simulink model "acc_PV"  (R2021b)
settings: Solver=FixedStepAuto  StartTime=0.0  StopTime=40  FixedStep=0.0005  RelTol=1e-3
undefined symbols (not defined in the file or in its folder): sigbuilder_block
libraries: Solver_SF x1
settings Model: Creator=power  LastModifiedBy=power
settings DataIOCC: ReturnWorkspaceOutputs=off

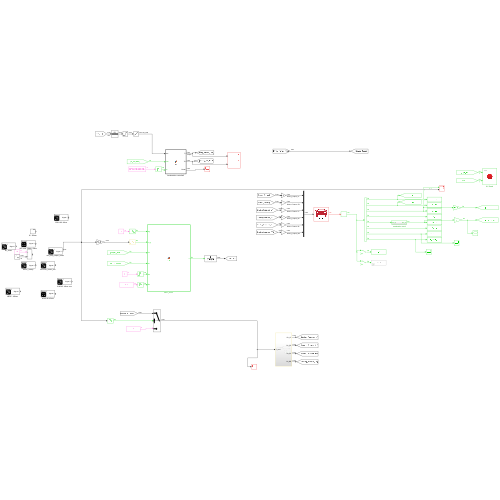
[thumbnail: Simulink's stored preview of the top-level diagram]
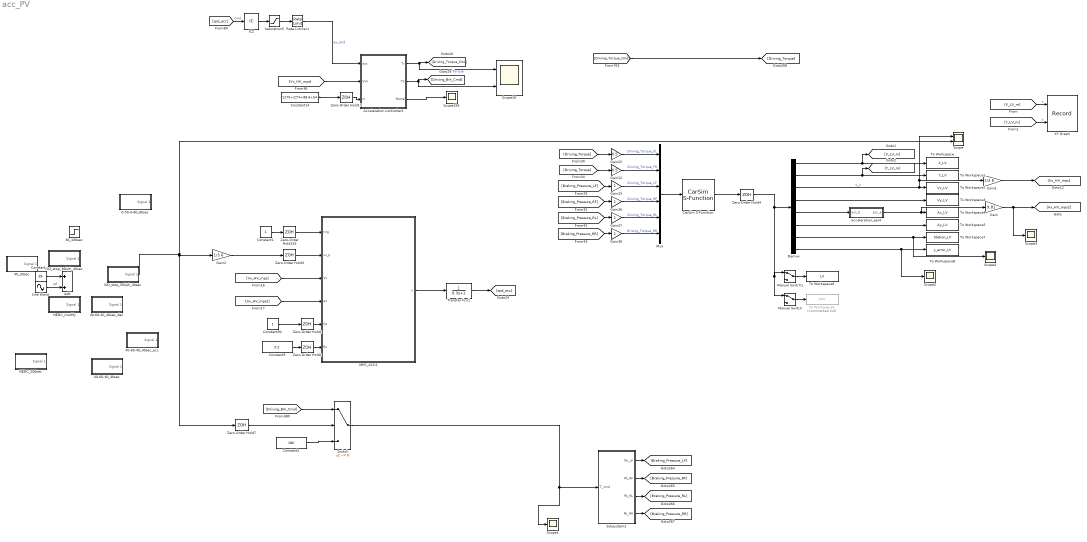
== system acc_PV ==
  0-50-0-80_80sec : Subsystem  Tag=STV Subsys  LoadFcn=sigbuilder_block('load');  StartFcn=sigbuilder_block('start');  StopFcn=sigbuilder_block('stop');  ClipboardFcn=sigbuilder_block('clipboard');  mask(Sigbuilder block){tuvar=[0:10]}
      mask help: Simulink:masks:SigbuilderBlock_MD
      mask init:
      | if ~strcmp(get_param(bdroot(gcbh),'SimulationStatus'),'stopped') tuvar = sigbuilder_block('maskInit'); end
      settings: CopyFcn=sigbuilder_block('copy');  DeleteFcn=sigbuilder_block('delete');  ModelCloseFcn=sigbuilder_block('modelClose');  PreSaveFcn=sigbuilder_block('preSave');  PauseFcn=sigbuilder_block('pause');  ContinueFcn=sigbuilder_block('continue');  NameChangeFcn=sigbuilder_block('namechange');  OpenFcn=sigbuilder_block('open',[523.8 -84 622.8 385.8 ]);  CloseFcn=sigbuilder_block('close');
      mask Display: plot(0, 0, 100, 100,[2, 2, 32, 32, 2], [68, 8, 8, 68, 68],[32, 2], [38, 38], [32, 19, 2],[53, 60, 44], [32, 17, 17, 2],[16, 16, 31, 31]);txt = getActiveGroup(gcbh);text(2, 100, txt,'verticalAlignment', 'top');
  36_100sec : Step  Time=0  Before=28  After=28  SampleTime=0
  40-60-40_40sec : Subsystem  Tag=STV Subsys  LoadFcn=sigbuilder_block('load');  StartFcn=sigbuilder_block('start');  StopFcn=sigbuilder_block('stop');  ClipboardFcn=sigbuilder_block('clipboard');  mask(Sigbuilder block){tuvar=[0:10]}
      mask help: Simulink:masks:SigbuilderBlock_MD
      mask init:
      | if ~strcmp(get_param(bdroot(gcbh),'SimulationStatus'),'stopped') tuvar = sigbuilder_block('maskInit'); end
      settings: CopyFcn=sigbuilder_block('copy');  DeleteFcn=sigbuilder_block('delete');  ModelCloseFcn=sigbuilder_block('modelClose');  PreSaveFcn=sigbuilder_block('preSave');  PauseFcn=sigbuilder_block('pause');  ContinueFcn=sigbuilder_block('continue');  NameChangeFcn=sigbuilder_block('namechange');  OpenFcn=sigbuilder_block('open',[595.8 96 550.8 208.2 ]);  CloseFcn=sigbuilder_block('close');
      mask Display: plot(0, 0, 100, 100,[2, 2, 32, 32, 2], [68, 8, 8, 68, 68],[32, 2], [38, 38], [32, 19, 2],[53, 60, 44], [32, 17, 17, 2],[16, 16, 31, 31]);txt = getActiveGroup(gcbh);text(2, 100, txt,'verticalAlignment', 'top');
  40-60-40_40sec_acc : Subsystem  Tag=STV Subsys  LoadFcn=sigbuilder_block('load');  StartFcn=sigbuilder_block('start');  StopFcn=sigbuilder_block('stop');  ClipboardFcn=sigbuilder_block('clipboard');  mask(Sigbuilder block){tuvar=[0:10]}
      mask help: Simulink:masks:SigbuilderBlock_MD
      mask init:
      | if ~strcmp(get_param(bdroot(gcbh),'SimulationStatus'),'stopped') tuvar = sigbuilder_block('maskInit'); end
      settings: CopyFcn=sigbuilder_block('copy');  DeleteFcn=sigbuilder_block('delete');  ModelCloseFcn=sigbuilder_block('modelClose');  PreSaveFcn=sigbuilder_block('preSave');  PauseFcn=sigbuilder_block('pause');  ContinueFcn=sigbuilder_block('continue');  NameChangeFcn=sigbuilder_block('namechange');  OpenFcn=sigbuilder_block('open',[595.8 79.8 550.8 169.8 ]);  CloseFcn=sigbuilder_block('close');
      mask Display: plot(0, 0, 100, 100,[2, 2, 32, 32, 2], [68, 8, 8, 68, 68],[32, 2], [38, 38], [32, 19, 2],[53, 60, 44], [32, 17, 17, 2],[16, 16, 31, 31]);txt = getActiveGroup(gcbh);text(2, 100, txt,'verticalAlignment', 'top');
  40-60-40_40sec_dec : Subsystem  Tag=STV Subsys  LoadFcn=sigbuilder_block('load');  StartFcn=sigbuilder_block('start');  StopFcn=sigbuilder_block('stop');  ClipboardFcn=sigbuilder_block('clipboard');  mask(Sigbuilder block){tuvar=[0:10]}
      mask help: Simulink:masks:SigbuilderBlock_MD
      mask init:
      | if ~strcmp(get_param(bdroot(gcbh),'SimulationStatus'),'stopped') tuvar = sigbuilder_block('maskInit'); end
      settings: CopyFcn=sigbuilder_block('copy');  DeleteFcn=sigbuilder_block('delete');  ModelCloseFcn=sigbuilder_block('modelClose');  PreSaveFcn=sigbuilder_block('preSave');  PauseFcn=sigbuilder_block('pause');  ContinueFcn=sigbuilder_block('continue');  NameChangeFcn=sigbuilder_block('namechange');  OpenFcn=sigbuilder_block('open',[2016 261.6 550.8 132.6 ]);  CloseFcn=sigbuilder_block('close');
      mask Display: plot(0, 0, 100, 100,[2, 2, 32, 32, 2], [68, 8, 8, 68, 68],[32, 2], [38, 38], [32, 19, 2],[53, 60, 44], [32, 17, 17, 2],[16, 16, 31, 31]);txt = getActiveGroup(gcbh);text(2, 100, txt,'verticalAlignment', 'top');
  40_30sec : Subsystem  Tag=STV Subsys  LoadFcn=sigbuilder_block('load');  StartFcn=sigbuilder_block('start');  StopFcn=sigbuilder_block('stop');  ClipboardFcn=sigbuilder_block('clipboard');  mask(Sigbuilder block){tuvar=[0:10]}
      mask help: Simulink:masks:SigbuilderBlock_MD
      mask init:
      | if ~strcmp(get_param(bdroot(gcbh),'SimulationStatus'),'stopped') tuvar = sigbuilder_block('maskInit'); end
      settings: CopyFcn=sigbuilder_block('copy');  DeleteFcn=sigbuilder_block('delete');  ModelCloseFcn=sigbuilder_block('modelClose');  PreSaveFcn=sigbuilder_block('preSave');  PauseFcn=sigbuilder_block('pause');  ContinueFcn=sigbuilder_block('continue');  NameChangeFcn=sigbuilder_block('namechange');  OpenFcn=sigbuilder_block('open',[595.8 -60 550.8 246.6 ]);  CloseFcn=sigbuilder_block('close');
      mask Display: plot(0, 0, 100, 100,[2, 2, 32, 32, 2], [68, 8, 8, 68, 68],[32, 2], [38, 38], [32, 19, 2],[53, 60, 44], [32, 17, 17, 2],[16, 16, 31, 31]);txt = getActiveGroup(gcbh);text(2, 100, txt,'verticalAlignment', 'top');
  Acceleration controller2 : MATLAB Function  TreatAsAtomicUnit=on
  Add : Sum
  CarSim S-Function : Solver_SF/CarSim S-Function  Priority=1  SIMFILE=simfile.sim  Run_RTs=off  vs_state_ind=Run  StopMode_ind=Vehicle Model
  Constant : Constant  Value=28
  Constant1 : Constant
  Constant14 : Constant  Value=1270+22*4+88.6+54.4
  Constant2 : Constant  Value=180
  Constant5 : Constant  Value=0.2
  Constant92 : Constant
  Demux : Demux  Outputs=8
  Gain : Gain  Gain=9.81
  Gain1 : Gain  Gain=1/3.6
  Gain12 : Gain  Gain=0.5
  Gain2 : Gain  Gain=1/3.6
  Gain22 : Gain  Gain=0.5
  Gain{33,36..38} (4 alike) : Gain
  IC2 : InitialCondition  Value=0
  ISO_stop_36kph_40sec : Subsystem  Tag=STV Subsys  LoadFcn=sigbuilder_block('load');  StartFcn=sigbuilder_block('start');  StopFcn=sigbuilder_block('stop');  ClipboardFcn=sigbuilder_block('clipboard');  mask(Sigbuilder block){tuvar=[0:10]}
      mask help: Simulink:masks:SigbuilderBlock_MD
      mask init:
      | if ~strcmp(get_param(bdroot(gcbh),'SimulationStatus'),'stopped') tuvar = sigbuilder_block('maskInit'); end
      settings: CopyFcn=sigbuilder_block('copy');  DeleteFcn=sigbuilder_block('delete');  ModelCloseFcn=sigbuilder_block('modelClose');  PreSaveFcn=sigbuilder_block('preSave');  PauseFcn=sigbuilder_block('pause');  ContinueFcn=sigbuilder_block('continue');  NameChangeFcn=sigbuilder_block('namechange');  OpenFcn=sigbuilder_block('open',[1635.6 28.8 550.8 208.2 ]);  CloseFcn=sigbuilder_block('close');
      mask Display: plot(0, 0, 100, 100,[2, 2, 32, 32, 2], [68, 8, 8, 68, 68],[32, 2], [38, 38], [32, 19, 2],[53, 60, 44], [32, 17, 17, 2],[16, 16, 31, 31]);txt = getActiveGroup(gcbh);text(2, 100, txt,'verticalAlignment', 'top');
  ISO_stop_50kph_40sec : Subsystem  Tag=STV Subsys  LoadFcn=sigbuilder_block('load');  StartFcn=sigbuilder_block('start');  StopFcn=sigbuilder_block('stop');  ClipboardFcn=sigbuilder_block('clipboard');  mask(Sigbuilder block){tuvar=[0:10]}
      mask help: Simulink:masks:SigbuilderBlock_MD
      mask init:
      | if ~strcmp(get_param(bdroot(gcbh),'SimulationStatus'),'stopped') tuvar = sigbuilder_block('maskInit'); end
      settings: CopyFcn=sigbuilder_block('copy');  DeleteFcn=sigbuilder_block('delete');  ModelCloseFcn=sigbuilder_block('modelClose');  PreSaveFcn=sigbuilder_block('preSave');  PauseFcn=sigbuilder_block('pause');  ContinueFcn=sigbuilder_block('continue');  NameChangeFcn=sigbuilder_block('namechange');  OpenFcn=sigbuilder_block('open',[455.25 155.25 590.25 348.75 ]);  CloseFcn=sigbuilder_block('close');
      mask Display: plot(0, 0, 100, 100,[2, 2, 32, 32, 2], [68, 8, 8, 68, 68],[32, 2], [38, 38], [32, 19, 2],[53, 60, 44], [32, 17, 17, 2],[16, 16, 31, 31]);txt = getActiveGroup(gcbh);text(2, 100, txt,'verticalAlignment', 'top');
  MPC_ACC2 : MATLAB Function  TreatAsAtomicUnit=on
  Manual Switch : ManualSwitch
  Manual Switch1 : ManualSwitch
  Mux : Mux  Inputs=6
  NEDC_206sec : Subsystem  Tag=STV Subsys  LoadFcn=sigbuilder_block('load');  StartFcn=sigbuilder_block('start');  StopFcn=sigbuilder_block('stop');  ClipboardFcn=sigbuilder_block('clipboard');  mask(Sigbuilder block){tuvar=[0:10]}
      mask help: Simulink:masks:SigbuilderBlock_MD
      mask init:
      | if ~strcmp(get_param(bdroot(gcbh),'SimulationStatus'),'stopped') tuvar = sigbuilder_block('maskInit'); end
      settings: CopyFcn=sigbuilder_block('copy');  DeleteFcn=sigbuilder_block('delete');  ModelCloseFcn=sigbuilder_block('modelClose');  PreSaveFcn=sigbuilder_block('preSave');  PauseFcn=sigbuilder_block('pause');  ContinueFcn=sigbuilder_block('continue');  NameChangeFcn=sigbuilder_block('namechange');  OpenFcn=sigbuilder_block('open',[5.4 107.4 1141.2 479.4 ]);  CloseFcn=sigbuilder_block('close');
      mask Display: plot(0, 0, 100, 100,[2, 2, 32, 32, 2], [68, 8, 8, 68, 68],[32, 2], [38, 38], [32, 19, 2],[53, 60, 44], [32, 17, 17, 2],[16, 16, 31, 31]);txt = getActiveGroup(gcbh);text(2, 100, txt,'verticalAlignment', 'top');
  NEDC_modify : Subsystem  Tag=STV Subsys  LoadFcn=sigbuilder_block('load');  StartFcn=sigbuilder_block('start');  StopFcn=sigbuilder_block('stop');  ClipboardFcn=sigbuilder_block('clipboard');  mask(Sigbuilder block){tuvar=[0:10]}
      mask help: Simulink:masks:SigbuilderBlock_MD
      mask init:
      | if ~strcmp(get_param(bdroot(gcbh),'SimulationStatus'),'stopped') tuvar = sigbuilder_block('maskInit'); end
      settings: CopyFcn=sigbuilder_block('copy');  DeleteFcn=sigbuilder_block('delete');  ModelCloseFcn=sigbuilder_block('modelClose');  PreSaveFcn=sigbuilder_block('preSave');  PauseFcn=sigbuilder_block('pause');  ContinueFcn=sigbuilder_block('continue');  NameChangeFcn=sigbuilder_block('namechange');  OpenFcn=sigbuilder_block('open',[5.4 87.6 1141.2 441 ]);  CloseFcn=sigbuilder_block('close');
      mask Display: plot(0, 0, 100, 100,[2, 2, 32, 32, 2], [68, 8, 8, 68, 68],[32, 2], [38, 38], [32, 19, 2],[53, 60, 44], [32, 17, 17, 2],[16, 16, 31, 31]);txt = getActiveGroup(gcbh);text(2, 100, txt,'verticalAlignment', 'top');
  Rate Limiter1 : RateLimiter  RisingSlewLimit=1.8  FallingSlewLimit=-1.8  SampleTimeMode=inherited
  Saturation5 : Saturate  UpperLimit=2  LowerLimit=-2
  Scope : Scope  NumInputPorts=2
  Scope{1..4,159} (5 alike) : Scope
  Scope16 : Scope  NumInputPorts=2
  Sine Wave : Sin  Amplitude=5  Frequency=0.5  SampleTime=0
  Subsystem2 : Subsystem
  Switch : Switch  Criteria=u2 ~= 0
  To Workspace : ToWorkspace  VariableName=X_LV  SampleTime=-1
  To Workspace1 : ToWorkspace  VariableName=Y_LV  SampleTime=-1
  To Workspace2 : ToWorkspace  VariableName=Vx_LV  SaveFormat=Timeseries  SampleTime=-1
  To Workspace3 : ToWorkspace  VariableName=Vy_LV  SampleTime=-1
  To Workspace4 : ToWorkspace  VariableName=Ax_LV  SampleTime=-1
  To Workspace5 : ToWorkspace  VariableName=Ay_LV  SampleTime=-1
  To Workspace6 : ToWorkspace  VariableName=LV  SaveFormat=Timeseries  SampleTime=-1
  To Workspace7 : ToWorkspace  VariableName=Station_LV  SampleTime=-1
  To Workspace8 : ToWorkspace  VariableName=y_error_LV  SampleTime=-1
  To Workspace9 : ToWorkspace  Commented=on  VariableName=APV  SaveFormat=Timeseries  SampleTime=-1
  Transfer Fcn1 : TransferFcn  Denominator=[0.3 1]
  XY Graph : Record  FileSettingsInternal="{\"entries\":[{\"content\":{\"excelSettings\":{\"content\":{},\"type\":\"Streamout.ExcelSettings\"}},\"type\":\"Streamout.FileSettingStorage\",\"uuid\":\"2b466944-9135-480b-8b79-00cf4fc90526\"}],\"packageUris\":[\"http://schema.mathworks.com/mf0/streamout_blocks/R2020a\"],\"version\":\"1.0\"}"  Layout=[1 1]  SignalsInternal="{\"entries\":[{\"content\":{\"signals\":[{\"content\":{\"blockPath\":[\"acc_PV/XY Graph\"],\"channel\":[],\"dimensions\":[1],\"domain\":\"acc_PV/XY Graph\",\"lineColor\":\"#a2142f\",\"plots\":[1],\"port\":1,\"sid\":[\"\"],\"signalID\":120332,\"signalName\":\"x\"},\"type\":\"RecordBlkView.Signal\",\"uuid\":\"004188c3-44d7-4870-b72c-abab145979a2\"},{\"content\":{\"blockPath\":[\"acc_PV/XY Graph\"],\"channel\":[],\"dimensions\":[1],\"domain\":\"acc_PV/XY Graph\",\"lineColor\":\"#139fff\",\"plots\":[1],\"port\":2,\"sid\":[\"\"],\"signalID\":120336,\"signalName\":\"y\"},\"type\":\"RecordBlkView.Signal\",\"uuid\":\"fd07caa7-1393-4bc3-b6a2-756354164627\"}]},\"type\":\"RecordBlkView.InputSignals\",\"uuid\":\"10821207-8221-4188-b325-d02c7d2ae950\"}],\"packageUris\":[\"http://schema.mathworks.com/mf0/streamout_blocks/R2020a\"],\"version\":\"1.0\"}"  VisualizationBindings="{\"xyplotplugin\":{\"info\":[{\"series\":[{\"bindingParametersList\":[{\"parameter\":\"X-Axis\",\"signalID\":120332,\"signalName\":\"x\"},{\"parameter\":\"Y-Axis\",\"signalID\":120336,\"signalName\":\"y\"}],\"seriesID\":48682}],\"subplotID\":1}]}}"  CompatibilityTag=XY
  Zero-Order Hold{1..4,7,17,133} (7 alike) : ZeroOrderHold  SampleTime=0.1
  acceleration_apr4 : Subsystem
  wires:
  Demux/1 -> [X_LV_m], To Workspace/1
  Demux/4 -> To Workspace3/1
  Demux/5 -> acceleration_apr4/1(acc_b)
  Demux/6 -> To Workspace5/1
  Mux/1 -> CarSim S-Function/1
  Zero-Order Hold133/1 -> MPC_ACC2/1(trig)
  Zero-Order Hold2/1 -> MPC_ACC2/6(Rs)
  Zero-Order Hold1/1 -> MPC_ACC2/5(Qs)
  Constant5/1 -> Zero-Order Hold2/1
  Constant92/1 -> Zero-Order Hold1/1
  MPC_ACC2/1(u) -> Transfer Fcn1/1
  Acceleration controller2/2(Tb) -> [Driving_Brk_Cmd], Scope16/2
  Rate Limiter1/1 -> Acceleration controller2/1(axc)  "ax_cmd"
  Constant14/1 -> Zero-Order Hold17/1
  Acceleration controller2/3(Rtotal) -> Scope159/1
  Acceleration controller2/1(Tr) -> [Driving_Torque_Cmd], Scope16/1  "Torque"
  Zero-Order Hold17/1 -> Acceleration controller2/3(m)
  Saturation5/1 -> Rate Limiter1/1
  IC2/1 -> Saturation5/1
  [spd_acc] -> IC2/1  "cmd"
  Gain12/1 -> Mux/2  "Driving_Torque_FR"
  [Driving_Torque] -> Gain12/1
  Gain22/1 -> Mux/1  "Driving_Torque_FL"
  [Driving_Torque] -> Gain22/1
  [Driving_Torque_Cmd] -> [Driving_Torque]
  Switch/1 -> Scope1/1, Subsystem2/1(T_cmd)
  Subsystem2/4(Pb_RR) -> [Braking_Pressure_RR]
  Subsystem2/1(Pb_LF) -> [Braking_Pressure_LF]
  Subsystem2/3(Pb_RL) -> [Braking_Pressure_RL]
  Subsystem2/2(Pb_RF) -> [Braking_Pressure_RF]
  [Braking_Pressure_LF] -> Gain33/1
  [Braking_Pressure_RF] -> Gain36/1
  [Braking_Pressure_RR] -> Gain38/1
  [Braking_Pressure_RL] -> Gain37/1
  Gain33/1 -> Mux/3  "Driving_Torque_LF"
  Gain36/1 -> Mux/4  "Driving_Torque_RF"
  Gain37/1 -> Mux/5  "Driving_Torque_RL"
  Gain38/1 -> Mux/6  "Driving_Torque_RR"
  Constant1/1 -> Zero-Order Hold133/1
  Zero-Order Hold3/1 -> MPC_ACC2/2(vx_p)
  [Driving_Brk_Cmd] -> Switch/1
  Constant2/1 -> Switch/3
  acceleration_apr4/1(acc_a) -> Gain/1, To Workspace4/1
  CarSim S-Function/1 -> Zero-Order Hold4/1
  [Ax_HV_mps2] -> MPC_ACC2/4(ax)
  [Vx_HV_mps] -> MPC_ACC2/3(Vx)
  [Vx_HV_mps] -> Acceleration controller2/2(Vxh)
  Zero-Order Hold7/1 -> Switch/2
  Sine Wave/1 -> Add/2  "ref"
  Gain/1 -> Scope3/1, [Ax_HV_mps2]
  Gain1/1 -> [Vx_HV_mps]
  Gain2/1 -> Zero-Order Hold3/1
  Zero-Order Hold4/1 -> Manual Switch1/1, Manual Switch/1, Demux/1
  Transfer Fcn1/1 -> [spd_acc]
  Demux/3 -> Scope/1, Gain1/1, To Workspace2/1  "V_x"
  Demux/7 -> Scope4/1, To Workspace7/1
  Demux/2 -> [Y_LV_m], To Workspace1/1
  [X_LV_m] -> XY Graph/1  "x"
  [Y_LV_m] -> XY Graph/2  "y"
  ISO_stop_50kph_40sec/1(Signal 1) -> Scope/2, Zero-Order Hold7/1, Gain2/1
  Constant/1 -> Add/1
  Demux/8 -> Scope2/1, To Workspace8/1
  Manual Switch1/1 -> To Workspace6/1
  Manual Switch/1 -> To Workspace9/1

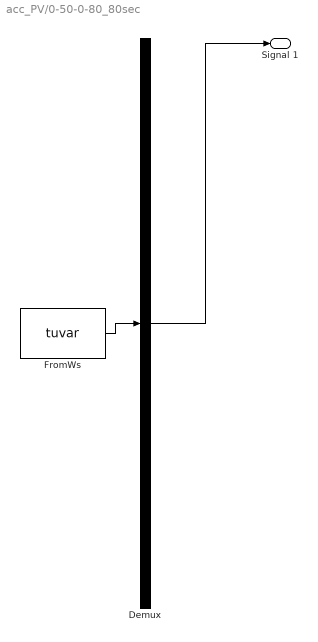
== system acc_PV/0-50-0-80_80sec ==
  Demux : Demux  Tag=STV Demux  Outputs=1
      settings: DisplayOption=none
  FromWs : FromWorkspace  Tag=STV FromWs  VariableName=tuvar
      SigBuilderData=|
      | common.afterFinalStr = 'Extrapolate'
      | common.sampleTime = 0
      | dataSet.timeRange = [0 80]
      | dataSet.name = 'Group 1'
      | sbobj.Groups.Name = 'Group 1'
      | sbobj.Groups.Signals.Name = 'Signal 1'
      | sbobj.Groups.Signals.XData = [0 10 20 30 35 45 55 65 80]
      | sbobj.Groups.Signals.YData = [0 50 50 0 0 60 60 0 0]
      | sbobj.Groups.TimeRange = [0 80]
  Signal 1 : Outport  Tag=STV Outport
  wires:
  FromWs/1 -> Demux/1
  Demux/1 -> Signal 1/1

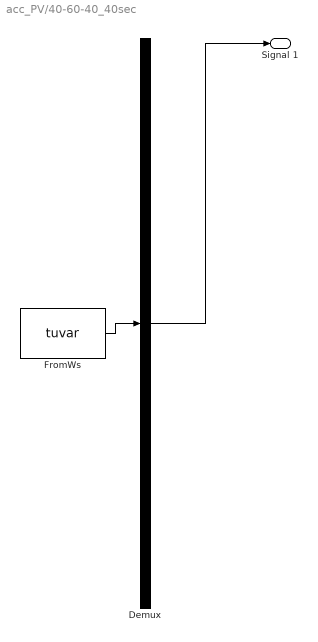
== system acc_PV/40-60-40_40sec ==
  Demux : Demux  Tag=STV Demux  Outputs=1
      settings: DisplayOption=none
  FromWs : FromWorkspace  Tag=STV FromWs  VariableName=tuvar
      SigBuilderData=|
      | common.afterFinalStr = 'Extrapolate'
      | common.sampleTime = 0
      | dataSet.timeRange = [0 40]
      | dataSet.name = 'Group 1'
      | sbobj.Groups.Name = 'Group 1'
      | sbobj.Groups.Signals.Name = 'Signal 1'
      | sbobj.Groups.Signals.XData = [0 10 20 30 40]
      | sbobj.Groups.Signals.YData = [40 60 60 40 40]
      | sbobj.Groups.TimeRange = [0 40]
  Signal 1 : Outport  Tag=STV Outport
  wires:
  FromWs/1 -> Demux/1
  Demux/1 -> Signal 1/1

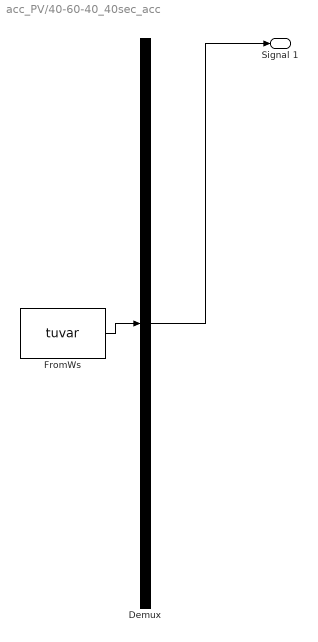
== system acc_PV/40-60-40_40sec_acc ==
  Demux : Demux  Tag=STV Demux  Outputs=1
      settings: DisplayOption=none
  FromWs : FromWorkspace  Tag=STV FromWs  VariableName=tuvar
      SigBuilderData=|
      | common.afterFinalStr = 'Extrapolate'
      | common.sampleTime = 0
      | dataSet.timeRange = [0 40]
      | dataSet.name = 'Group 1'
      | sbobj.Groups.Name = 'Group 1'
      | sbobj.Groups.Signals.Name = 'Signal 1'
      | sbobj.Groups.Signals.XData = [0 10 15.5 16 18 18.5 20 25 40]
      | sbobj.Groups.Signals.YData = [40 60 60 62 62 60 60 40 40]
      | sbobj.Groups.TimeRange = [0 40]
  Signal 1 : Outport  Tag=STV Outport
  wires:
  Demux/1 -> Signal 1/1
  FromWs/1 -> Demux/1

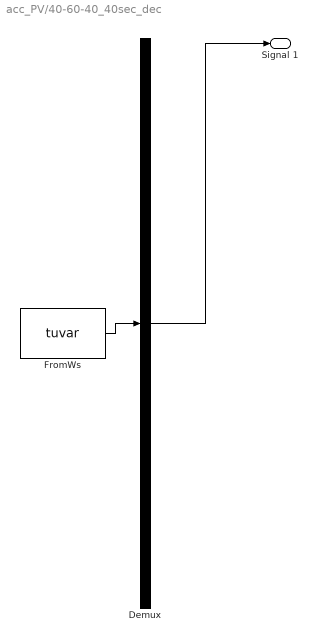
== system acc_PV/40-60-40_40sec_dec ==
  Demux : Demux  Tag=STV Demux  Outputs=1
      settings: DisplayOption=none
  FromWs : FromWorkspace  Tag=STV FromWs  VariableName=tuvar
      SigBuilderData=|
      | common.afterFinalStr = 'Extrapolate'
      | common.sampleTime = 0
      | dataSet.timeRange = [0 40]
      | dataSet.name = 'Group 1'
      | sbobj.Groups.Name = 'Group 1'
      | sbobj.Groups.Signals.Name = 'Signal 1'
      | sbobj.Groups.Signals.XData = [0 10 15.5 16 18 18.5 20 25 40]
      | sbobj.Groups.Signals.YData = [40 60 60 50 50 60 60 40 40]
      | sbobj.Groups.TimeRange = [0 40]
  Signal 1 : Outport  Tag=STV Outport
  wires:
  FromWs/1 -> Demux/1
  Demux/1 -> Signal 1/1

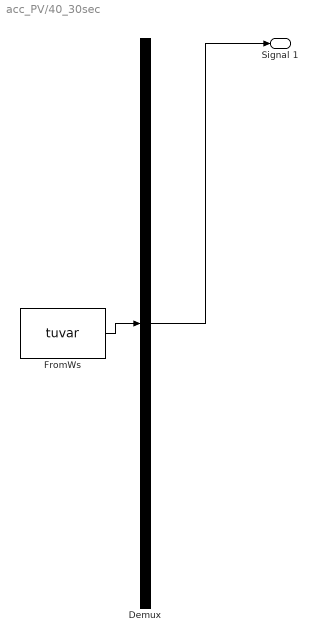
== system acc_PV/40_30sec ==
  Demux : Demux  Tag=STV Demux  Outputs=1
      settings: DisplayOption=none
  FromWs : FromWorkspace  Tag=STV FromWs  VariableName=tuvar
      SigBuilderData=|
      | common.afterFinalStr = 'Extrapolate'
      | common.sampleTime = 0
      | dataSet.timeRange = [0 30]
      | dataSet.name = 'Group 1'
      | sbobj.Groups.Name = 'Group 1'
      | sbobj.Groups.Signals.Name = 'Signal 1'
      | sbobj.Groups.Signals.XData = [0 10 20 30]
      | sbobj.Groups.Signals.YData = [40 40 40 40]
      | sbobj.Groups.TimeRange = [0 30]
  Signal 1 : Outport  Tag=STV Outport
  wires:
  Demux/1 -> Signal 1/1
  FromWs/1 -> Demux/1

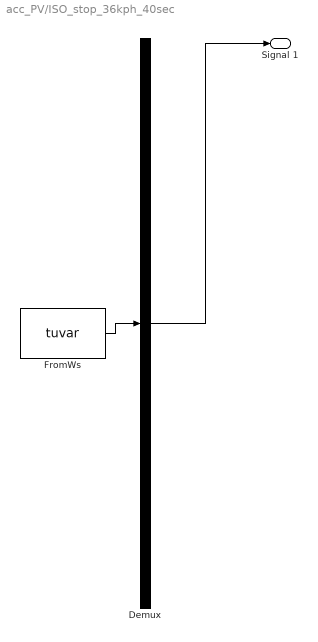
== system acc_PV/ISO_stop_36kph_40sec ==
  Demux : Demux  Tag=STV Demux  Outputs=1
      settings: DisplayOption=none
  FromWs : FromWorkspace  Tag=STV FromWs  VariableName=tuvar
      SigBuilderData=|
      | common.afterFinalStr = 'Extrapolate'
      | common.sampleTime = 0
      | dataSet.timeRange = [0 40]
      | dataSet.name = 'Group 1'
      | sbobj.Groups.Name = 'Group 1'
      | sbobj.Groups.Signals.Name = 'Signal 1'
      | sbobj.Groups.Signals.XData = [0 10 20 24 40]
      | sbobj.Groups.Signals.YData = [36 36 36 0 0]
      | sbobj.Groups.TimeRange = [0 40]
  Signal 1 : Outport  Tag=STV Outport
  wires:
  Demux/1 -> Signal 1/1
  FromWs/1 -> Demux/1

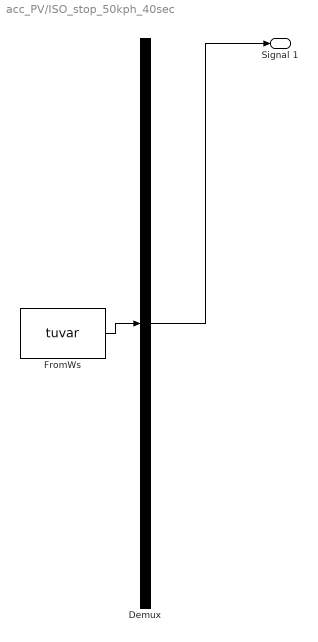
== system acc_PV/ISO_stop_50kph_40sec ==
  Demux : Demux  Tag=STV Demux  Outputs=1
      settings: DisplayOption=none
  FromWs : FromWorkspace  Tag=STV FromWs  VariableName=tuvar
      SigBuilderData=|
      | common.afterFinalStr = 'Extrapolate'
      | common.sampleTime = 0
      | dataSet.timeRange = [0 40]
      | dataSet.name = 'Group 1'
      | sbobj.Groups.Name = 'Group 1'
      | sbobj.Groups.Signals.Name = 'Signal 1'
      | sbobj.Groups.Signals.XData = [0 20 25.55 40]
      | sbobj.Groups.Signals.YData = [50 50 0 0]
      | sbobj.Groups.TimeRange = [0 40]
  Signal 1 : Outport  Tag=STV Outport
  wires:
  FromWs/1 -> Demux/1
  Demux/1 -> Signal 1/1

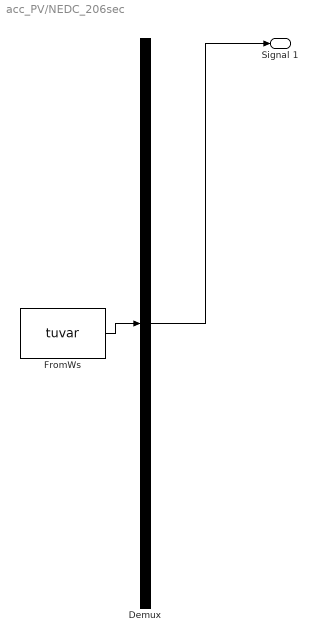
== system acc_PV/NEDC_206sec ==
  Demux : Demux  Tag=STV Demux  Outputs=1
      settings: DisplayOption=none
  FromWs : FromWorkspace  Tag=STV FromWs  VariableName=tuvar
      SigBuilderData=|
      | common.afterFinalStr = 'Extrapolate'
      | common.sampleTime = 0
      | dataSet.timeRange = [0 1200]
      | dataSet.name = 'Group 1'
      | sbobj.Groups.Name = 'Group 1'
      | sbobj.Groups.Signals.Name = 'Signal 1'
      | sbobj.Groups.Signals.XData = [0 11 15 23 28 49 61 85 96 117 143 155 163 176 188 195 206 210 218 223 244 256 280 291 312 338 350 358 371 383 390 401 405 413 418 439 451 475 486 507 533 545 553 566 578 585 596 600 608 613 634 646 670 681 702 728 740 748 761 773 780 800 841 891 899 968 981 1031 1066 1096 1116 1126 1160 1200]
      | sbobj.Groups.Signals.YData = [0 0 15 15 0 0 32 32 0 0 50 50 35 35 0 0 0 15 15 0 0 32 32 0 0 50 50 35 35 0 0 0 15 15 0 0 32 32 0 0 50 50 35 35 0 0 0 15 15 0 0 32 32 0 0 50 50 35 35 0 0 0 70 70 50 50 70 70 100 100 120 120 0 0]
      | sbobj.Groups.TimeRange = [0 1200]
  Signal 1 : Outport  Tag=STV Outport
  wires:
  FromWs/1 -> Demux/1
  Demux/1 -> Signal 1/1

== system acc_PV/NEDC_modify ==
  Demux : Demux  Tag=STV Demux  Outputs=1
      settings: DisplayOption=none
  FromWs : FromWorkspace  Tag=STV FromWs  VariableName=tuvar
      SigBuilderData=|
      | common.afterFinalStr = 'Extrapolate'
      | common.sampleTime = 0
      | dataSet.timeRange = [0 1200]
      | dataSet.name = 'Group 1'
      | sbobj.Groups.Name = 'Group 1'
      | sbobj.Groups.Signals.Name = 'Signal 1'
      | sbobj.Groups.Signals.XData = [0 11 15 23 28 49 61 85 96 117 143 155 163 176 188 195 206 210 218 223 244 256 280 291 312 338 350 358 371 383 390 401 405 413 418 439 451 475 486 507 533 545 553 566 578 585 596 600 608 613 634 646 670 681 702 728 740 748 761 773 780 800 841 891 899 968 981 1031 1066 1096 1116 1126 1160 1200]
      | sbobj.Groups.Signals.YData = [15 15 15 15 0 0 32 32 0 0 50 50 35 35 0 0 0 15 15 0 0 32 32 0 0 50 50 35 35 0 0 0 15 15 0 0 32 32 0 0 50 50 35 35 0 0 0 15 15 0 0 32 32 0 0 50 50 35 35 0 0 0 70 70 50 50 70 70 100 100 120 120 0 0]
      | sbobj.Groups.TimeRange = [0 1200]
  Signal 1 : Outport  Tag=STV Outport
  wires:
  Demux/1 -> Signal 1/1
  FromWs/1 -> Demux/1

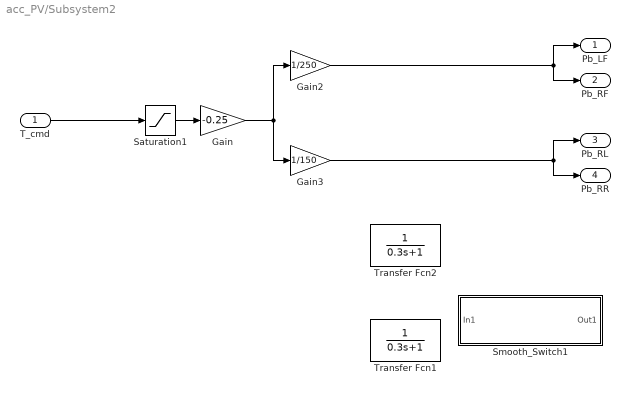
== system acc_PV/Subsystem2 ==
  T_cmd : Inport
  Gain : Gain  Gain=-0.25
  Gain2 : Gain  Gain=1/250
  Gain3 : Gain  Gain=1/150
  Saturation1 : Saturate  UpperLimit=0  LowerLimit=-inf
  Smooth_Switch1 : Subsystem  mask{tau=0.3, IC=0, T=0.1}
      mask prompts: tau "Time constant"; T "Sample time"
      mask Display:
      | fprintf('Discrete first order \n\n')
      | fprintf(['tau=' num2str(tau) '    IC=' num2str(IC)])
  Transfer Fcn1 : TransferFcn  Denominator=[0.3 1]
  Transfer Fcn2 : TransferFcn  Denominator=[0.3 1]
  Pb_LF : Outport
  Pb_RF : Outport  Port=2
  Pb_RL : Outport  Port=3
  Pb_RR : Outport  Port=4
  wires:
  Gain3/1 -> Pb_RR/1, Pb_RL/1
  Gain2/1 -> Pb_RF/1, Pb_LF/1
  Gain/1 -> Gain2/1, Gain3/1
  Saturation1/1 -> Gain/1
  T_cmd/1 -> Saturation1/1

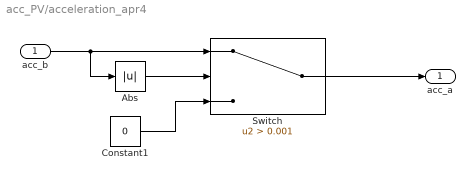
== system acc_PV/acceleration_apr4 ==
  acc_b : Inport
  Abs : Abs
  Constant1 : Constant  Value=0
  Switch : Switch  Criteria=u2 > Threshold  Threshold=0.001
  acc_a : Outport  VectorParamsAs1DForOutWhenUnconnected=off
  wires:
  Abs/1 -> Switch/2
  Constant1/1 -> Switch/3
  acc_b/1 -> Switch/1, Abs/1
  Switch/1 -> acc_a/1

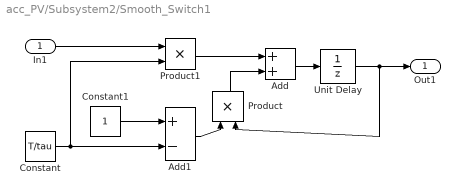
== system acc_PV/Subsystem2/Smooth_Switch1 ==
  In1 : Inport
  Add : Sum
  Add1 : Sum  Inputs=+-
  Constant : Constant  Value=T/tau
  Constant1 : Constant
  Product : Product
  Product1 : Product
  Unit Delay : UnitDelay  InitialCondition=IC  SampleTime=T  HasFrameUpgradeWarning=on
  Out1 : Outport
  wires:
  Constant1/1 -> Add1/1
  Constant/1 -> Add1/2, Product1/2
  Add1/1 -> Product/1
  In1/1 -> Product1/1
  Product/1 -> Add/2
  Unit Delay/1 -> Product/2, Out1/1
  Add/1 -> Unit Delay/1
  Product1/1 -> Add/1

== matlab function acc_PV/Acceleration controller2 ==
  data: axc input; Tr output; Vxh input; Tb output; Rtotal output; m input
function [Tr,Tb,Rtotal]= fcn(axc, Vxh,m)
% m_hat = 1370+89.9+65.2+22*4; 
m_hat = m;
Cd_hat = 0.3;     %Aerodynamic Coefficient
fr_hat = 0.0038;  %Rolling Resistance Moment

zho = 1.206;  %Air Mass density
Af = 2.2; %Front Area
g = 9.81;
rw = 0.325; %Effective rolling radius 

% m_hat = 1/theta_hat(1);
% Cd_hat = theta_hat(2)*m_hat;
% fr_hat = theta_hat(3);

theta = 0;
% Resistance

Ra = 0.5*zho*Cd_hat*Af*Vxh^2;
Rg = m_hat*g*sin(theta);
Rr = fr_hat*m_hat*g*cos(theta);
Rtotal = (Ra + Rg + Rr)*rw;

% if Vxh<1
%     Ra=0;
%     Rg=0;
%     Rr=0;
%     Rtotal =0;
% else
%     Ra = 0.5*zho*Cd_hat*Af*Vxh^2;
%     Rg = m_hat*g*sin(theta);
%     Rr = fr_hat*m_hat*g*cos(theta);
%     Rtotal = (Ra + Rg + Rr)*rw;
% end

Tr = (m_hat*axc + Ra + Rg + Rr)*rw;
Tb = (m_hat*axc - Ra - Rg - Rr)*rw;

% if axc >= 0
%     Tr = Tr;
%     Tb = 0;
% else
%     Tr = 0;
%     Tb = Tb;
% end

== matlab function acc_PV/MPC_ACC2 ==
  data: trig input; vx_p input; u output; Vx input; ax input; Qs input; Rs input
function u = fcn(trig,vx_p,Vx,ax,Qs,Rs)
%% Initialzization
T = 0.1;
tau = 0.3;
Np = 10;
Nc = 3;

%% Mode Selector && MPC

A_spd = [1 T;0 1-T/tau];
B_spd = [0;T/tau];
C_spd = [1 0];

if trig == 1
    [m1,n1] = size(C_spd);
    h = zeros(Np,n1);
    F = zeros(Np,n1);
    h(1,:)=C_spd;
    F(1,:)=C_spd*A_spd;
    for j=2:Np
    h(j,:)=h(j-1,:)*A_spd; %Phi
    F(j,:)= F(j-1,:)*A_spd; 
    end
    v = h*B_spd;
    Phi_vx = zeros(Np,Nc);
    Phi_vx(:,1) = v;
    for k = 2:Nc
       Phi_vx(:,k) = [zeros(k-1,1);v(1:Np-k+1,1)]; %Toeplitz matrix
    end
    Q=Qs.*eye(Np); %Qw權重值=1;10
    R=Rs.*eye(Nc);%Rw權重值=0.07;1.5 ,0.07
    
    x_spd = [Vx;ax];
    Yref = vx_p';
    
    H = Phi_vx'*Q*Phi_vx+R;
    f = Phi_vx'*Q*(Yref-F*x_spd);
    U = inv(H)*f;
    u = U(1);

else
    u=0;
end
end
